simulink subsystem "in_wave"  (R2025b)
settings: Solver=VariableStepAuto  StartTime=0.0  StopTime=10.0  RelTol=1e-3
settings Model: Creator=sanborkl  LastModifiedBy=admin

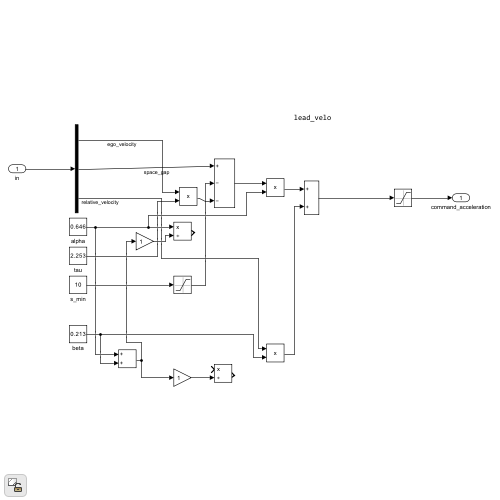
[thumbnail: Simulink's stored preview of the top-level diagram]
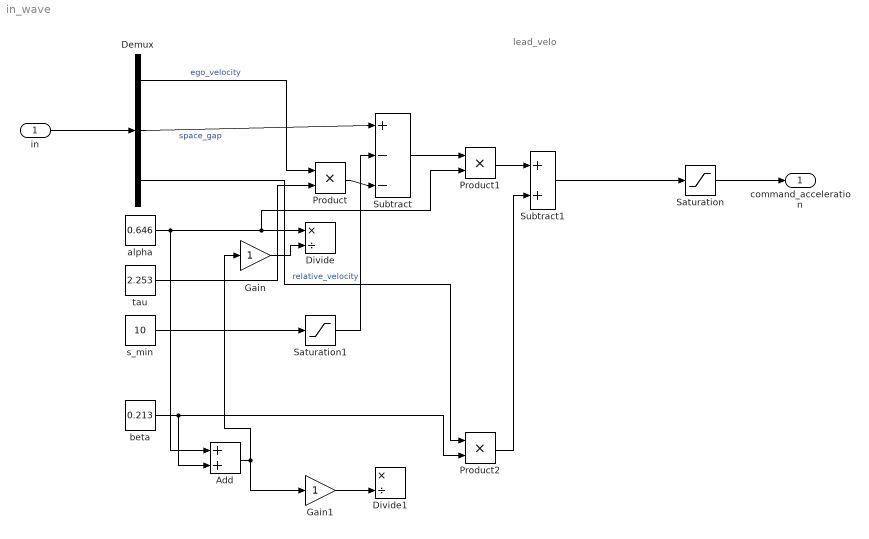
== system in_wave ==
  note: lead_velo
  in : Inport
  Add : Sum
  Demux : Demux  Outputs=3
  Divide : Product  Inputs=*/
  Divide1 : Product  Inputs=*/
  Gain : Gain
  Gain1 : Gain
  Product : Product
  Product1 : Product
  Product2 : Product
  Saturation : Saturate  UpperLimit=1.5  LowerLimit=-3.0
  Saturation1 : Saturate  UpperLimit=500  LowerLimit=2
  Subtract : Sum  Inputs=+--
  Subtract1 : Sum
  alpha : Constant  Value=0.646
  beta : Constant  Value=0.213
  s_min : Constant  Value=10
  tau : Constant  Value=2.253
  command_acceleration : Outport
  wires:
  alpha/1 -> Product1/2, Divide/1, Add/1
  tau/1 -> Product/2
  in/1 -> Demux/1
  Demux/1 -> Product/1  "ego_velocity"
  Demux/2 -> Subtract/1  "space_gap"
  Saturation/1 -> command_acceleration/1
  s_min/1 -> Saturation1/1
  Product/1 -> Subtract/3
  Subtract/1 -> Product1/1
  Product1/1 -> Subtract1/1
  Saturation1/1 -> Subtract/2
  beta/1 -> Product2/2, Add/2
  Demux/3 -> Product2/1  "relative_velocity"
  Subtract1/1 -> Saturation/1
  Gain/1 -> Divide/2
  Add/1 -> Gain1/1, Gain/1
  Gain1/1 -> Divide1/2
  Product2/1 -> Subtract1/2
